simulink model "kalman"  (R2020a)
settings: Solver=VariableStepAuto  StartTime=0.0  StopTime=100  MaxStep=0.01  MinStep=0.01  RelTol=1e-3
model workspace (MAT data in the model file):
  PnFrequencyOffset_26 = [30000 100000 1000000 3000000 10000000]
  uniqueString_26 = '91_3376'
libraries: simulink x1
settings Model: Creator=johan  LastModifiedBy=johan
settings DebuggingCC: UnconnectedInputMsg=none  UnconnectedOutputMsg=none  UnconnectedLineMsg=none
settings ModelReferenceCC: EnableRefExpFcnMdlSchedulingChecks=off
settings RTWCC: Description=Generic Real-Time Target

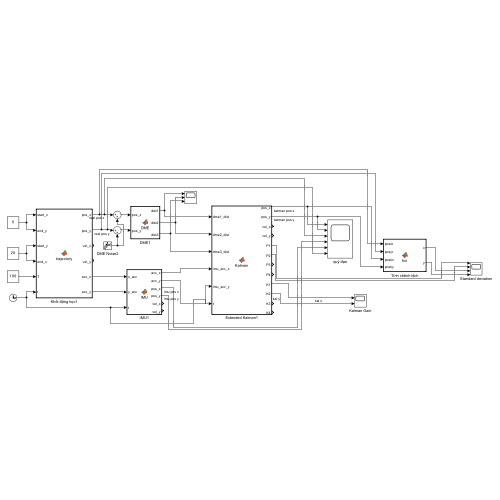
[thumbnail: Simulink's stored preview of the top-level diagram]
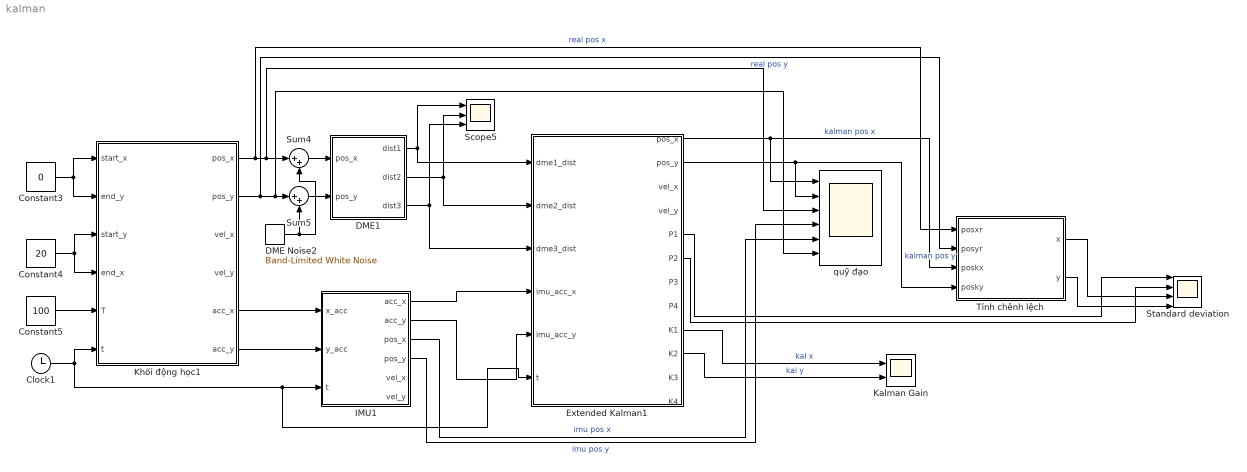
== system kalman ==
  Clock1 : Clock
  Constant3 : Constant  Value=0
  Constant4 : Constant  Value=20
  Constant5 : Constant  Value=100
  DME Noise2 : simulink/Sources/Band-Limited White Noise  Cov=[1e-5]  Ts=0.01  seed=[23341]
  DME1 : MATLAB Function  TreatAsAtomicUnit=on
  Extended Kalman1 : MATLAB Function  TreatAsAtomicUnit=on
  IMU1 : MATLAB Function  TreatAsAtomicUnit=on
  Kalman Gain : Scope  NumInputPorts=2
  Khối động học1 : MATLAB Function  TreatAsAtomicUnit=on
  Scope5 : Scope  NumInputPorts=3
  Standard deviation : Scope  NumInputPorts=4
  Sum4 : Sum  Inputs=|++
  Sum5 : Sum  Inputs=|++
  Tính chênh lệch : MATLAB Function  TreatAsAtomicUnit=on
  quỹ đạo : Scope  NumInputPorts=6
  wires:
  Extended Kalman1/2(pos_y) -> Tính chênh lệch/4(posky), quỹ đạo/2  "kalman pos y"
  Extended Kalman1/1(pos_x) -> Tính chênh lệch/3(poskx), quỹ đạo/1  "kalman pos x"
  Khối động học1/5(acc_x) -> IMU1/1(x_acc)
  IMU1/2(acc_y) -> Extended Kalman1/5(imu_acc_y)
  IMU1/1(acc_x) -> Extended Kalman1/4(imu_acc_x)
  DME1/1(dist1) -> Scope5/1, Extended Kalman1/1(dme1_dist)
  Khối động học1/6(acc_y) -> IMU1/2(y_acc)
  DME1/3(dist3) -> Extended Kalman1/3(dme3_dist), Scope5/3
  DME1/2(dist2) -> Extended Kalman1/2(dme2_dist), Scope5/2
  Constant4/1 -> Khối động học1/3(start_y), Khối động học1/4(end_x)
  Constant5/1 -> Khối động học1/5(T)
  Constant3/1 -> Khối động học1/2(end_y), Khối động học1/1(start_x)
  Clock1/1 -> IMU1/3(t), Extended Kalman1/6(t), Khối động học1/6(t)
  Sum5/1 -> DME1/2(pos_y)
  Sum4/1 -> DME1/1(pos_x)
  DME Noise2/1 -> Sum4/2, Sum5/2
  Khối động học1/2(pos_y) -> Tính chênh lệch/2(posyr), Sum5/1, quỹ đạo/6  "real pos y"
  Khối động học1/1(pos_x) -> Tính chênh lệch/1(posxr), Sum4/1, quỹ đạo/3  "real pos x"
  Extended Kalman1/5(P1) -> Standard deviation/1
  Extended Kalman1/6(P2) -> Standard deviation/2
  IMU1/3(pos_x) -> quỹ đạo/5  "imu pos x"
  IMU1/4(pos_y) -> quỹ đạo/4  "imu pos y"
  Extended Kalman1/9(K1) -> Kalman Gain/1  "kal x"
  Extended Kalman1/10(K2) -> Kalman Gain/2  "kal y"
  Tính chênh lệch/2(y) -> Standard deviation/4
  Tính chênh lệch/1(x) -> Standard deviation/3

== matlab function kalman/Tính chênh lệch ==
  data: x output; posxr input; y output; posyr input; poskx input; posky input
function [x,y] = fcn(posxr, posyr, poskx, posky)
x = abs(posxr-poskx);
y=abs(posyr-posky);

== matlab function kalman/DME1 ==
  data: pos_x input; dist1 output; pos_y input; dist2 output; dist3 output
function [dist1, dist2, dist3] = DME(pos_x, pos_y)
    % Define DME station positions
    dme1_x = 0; dme1_y = 22;     % Position of DME station 1
    dme2_x = 16; dme2_y = 16;      % Position of DME station 2
    dme3_x = 230; dme3_y = 100;     % Position of DME station 3
    
    % Define DME coverage radius
    coverage_radius = 7;
    % Calculate distances to each DME station
    dx1 = pos_x - dme1_x;
    dy1 = pos_y - dme1_y;
    range1 = sqrt(dx1^2 + dy1^2);
    if range1 <= coverage_radius
        dist1 = range1;
    else
        dist1 = NaN;
    end
    
    dx2 = pos_x - dme2_x;
    dy2 = pos_y - dme2_y;
    range2 = sqrt(dx2^2 + dy2^2);
    if range2 <= coverage_radius;
        dist2 = range2;
    else
        dist2 = NaN;
    end
    
    dx3 = pos_x - dme3_x;
    dy3 = pos_y - dme3_y;
    range3 = sqrt(dx3^2 + dy3^2);
    if range3 <= coverage_radius
        dist3 = range3;
    else
        dist3 = NaN;
    end
end

== matlab function kalman/Extended Kalman1 ==
  data: dme1_dist input; dme2_dist input; dme3_dist input; imu_acc_x input; imu_acc_y input; t input; pos_x output; pos_y output; vel_x output; vel_y output; P1 output; P2 output; P3 output; P4 output; K1 output; K2 output; K3 output; K4 output
function [pos_x, pos_y, vel_x, vel_y, P1, P2, P3, P4, K1, K2, K3, K4] = Kalman(dme1_dist, dme2_dist, dme3_dist, imu_acc_x, imu_acc_y, t)

    persistent x_est P_est prev_t
    if isempty(x_est)
        % Initialize state vector [pos_x; pos_y; vel_x; vel_y]
        x_est = [0; 20; 0; 0];  % Initial position 
        P_est = eye(4) * 1e-30;      % Initial state covariance
        prev_t = 0;
    end
    
    % Calculate dt
    dt = t - prev_t;
    prev_t = t; 
    a=2e-5;
    b=1.9e-5;
    c = 0;
    % Process noise covariance (Q)
    Q = [a	c  0	0;
          c   b	  0	0;
            0	        0	      0	0;
            0          0	      0	0];  
    
    R_single = 9.8e-04;  % Measurement noise variance
    
    % DME station positions
    dme1_pos = [0, 22];   % DME 1
    dme2_pos = [16, 16];  % DME 2
    dme3_pos = [23, 0];  % DME 3
    
    % Prediction Step
    % State transition matrix (F)
    F = [1, 0, dt, 0;
         0, 1, 0, dt;
         0, 0, 1, 0;
         0, 0, 0, 1];
    
    % Input matrix (B) for acceleration
    B = [0.5*dt^2, 0;
         0, 0.5*dt^2;
         dt, 0;
         0, dt];
    
    % Predict state
    x_pred = F * x_est + B * [imu_acc_x; imu_acc_y];
    
    % Predict covariance
    P_pred = F * P_est * F' + Q;
    
    % Update Step
    % Initialize measurement matrices
    H = zeros(1, 4);  % Single measurement, 4 states
    z = 0;            % Valid measurement
    h_x = 0;          % Predicted measurement
    R = 0;            % Measurement noise covariance
    
    % Check DME 1
    if dme1_dist > 0  % Valid measurement
        dx = x_pred(1) - dme1_pos(1);
        dy = x_pred(2) - dme1_pos(2);
        dist = sqrt(dx^2 + dy^2);
        
        % Populate H, z, h_x, and R for DME 1
        H = [dx/dist, dy/dist, 0, 0];
        z = dme1_dist;
        h_x = dist;
        R = R_single;
    end
    
    % Check DME 2
    if dme2_dist > 0  % Valid measurement
        dx = x_pred(1) - dme2_pos(1);
        dy = x_pred(2) - dme2_pos(2);
        dist = sqrt(dx^2 + dy^2);
        
        % Populate H, z, h_x, and R for DME 2
        H = [dx/dist, dy/dist, 0, 0];
        z = dme2_dist;
        h_x = dist;
        R = R_single;
    end
    
    % Check DME 3
    if dme3_dist > 0  % Valid measurement
        dx = x_pred(1) - dme3_pos(1);
        dy = x_pred(2) - dme3_pos(2);
        dist = sqrt(dx^2 + dy^2);
        
        % Populate H, z, h_x, and R for DME 3
        H = [dx/dist, dy/dist, 0, 0];
        z = dme3_dist;
        h_x = dist;
        R = R_single;
    end
    
    % Update state if we have a valid measurement
    if R > 0
        % Calculate Kalman gain
        S = H * P_pred * H' + R;
        K = P_pred * H' / S;
        
        % Extract components of Kalman gain
        K1 = K(1);
        K2 = K(2);
        K3 = K(3);
        K4 = K(4);
        
        % Update state and covariance
        residual = z - h_x;
        x_est = x_pred + K * residual;
        P_est = (eye(4) - K * H) * P_pred;
    else
        % If no valid measurements, use prediction
        x_est = x_pred;
        P_est = P_pred;
        K1 = 0;
        K2 = 0;
        K3 = 0;
        K4 = 0;
    end
        P1 = sqrt(P_est(1,1));
        P2 = sqrt(P_est(2,2));
            P3 = sqrt(P_est(3,3));
                P4 = sqrt(P_est(4,4));
    % Output estimated states and Kalman gain components
    pos_x = x_est(1);
    pos_y = x_est(2);
    vel_x = x_est(3);
    vel_y = x_est(4);
end

== matlab function kalman/IMU1 ==
  data: acc_x output; acc_y output; x_acc input; pos_x output; y_acc input; t input; pos_y output; vel_x output; vel_y output
function [ acc_x, acc_y,pos_x, pos_y, vel_x, vel_y] = IMU(x_acc, y_acc, t)
    g = 9.81;  % gravity constant [m/s^2]
    persistent prev_vel_x prev_vel_y prev_pos_x prev_pos_y prev_t
   
    if isempty(prev_vel_x)
        prev_vel_x = 0;
        prev_vel_y = 0;
        prev_pos_x = 0;  % Set to match trajectory starting position
        prev_pos_y = 20;  % Set to match trajectory starting position
        prev_t = 0;
    end
    
    % Calculate dt
    dt = t - prev_t;
    
    % Error parameters
    acc_bias_mps2 = 1e-5 * 9.81;  % accelerometer bias
    gyro_bias_rps = 1e-3 * (pi/180) / 3600;  % gyroscope bias
    init_heading_error_rad =1e-5 * (pi/180);  % heading error
    init_velocity_error = 0;  % velocity error
    init_position_error = 0;  % position error
    
    % Calculate errors 
    delta_theta = init_heading_error_rad + gyro_bias_rps * t;
    
    delta_v = init_velocity_error + acc_bias_mps2 * t - ...
              g * init_heading_error_rad * t - ...
              g * gyro_bias_rps * t^2;
    
    delta_p = init_position_error + init_velocity_error * t + ...
              0.5 * acc_bias_mps2 * t^2 - ...
              0.5 * g * init_heading_error_rad * t^2 - ...
              (1/6) * g * gyro_bias_rps * t^3;
    
    % Add bias to accelerometer readings
    acc_x = x_acc + acc_bias_mps2;
    acc_y = y_acc + acc_bias_mps2;
    
    % Integrate acceleration to get velocity
    vel_x = prev_vel_x + acc_x * dt;
    vel_y = prev_vel_y + acc_y * dt;
    
    % Add velocity error
    vel_x = vel_x + delta_v;
    vel_y = vel_y + delta_v;
    
    % Integrate velocity to get position
    pos_x = prev_pos_x + prev_vel_x * dt + 0.5 * acc_x * dt * dt;  
    pos_y = prev_pos_y + prev_vel_y * dt + 0.5 * acc_y * dt * dt;
    
    % Add position error
    pos_x = pos_x + delta_p;
    pos_y = pos_y + delta_p;
    
    % Update persistent variables
    prev_vel_x = vel_x - delta_v;
    prev_vel_y = vel_y - delta_v;
    prev_pos_x = pos_x - delta_p;
    prev_pos_y = pos_y - delta_p;
    prev_t = t;

end

== matlab function kalman/Khối động học1 ==
  data: start_x input; end_y input; start_y input; end_x input; T input; t input; pos_x output; pos_y output; vel_x output; vel_y output; acc_x output; acc_y output
function [pos_x, pos_y, vel_x, vel_y, acc_x, acc_y] = trajectory( start_x, end_y, start_y, end_x, T,t)
    % Normalize time to [0,1]
    t_norm = t/T;
    if t_norm > 1
        t_norm = 1;
    end
    
% X-direction
a0 = 0; a1 = 0; a2 = 0; a3 = 10; a4 = -15; a5 = 6;
% Y-direction
b0 = 0; b1 = 0; b2 = 0; b3 = 9; b4 = -18; b5 = 10;

    % Calculate normalized position 
    s = a0 + a1*t_norm + a2*t_norm^2 + a3*t_norm^3 + a4*t_norm^4 + a5*t_norm^5;
    
    % Calculate normalized velocity
    s_dot = (a1 + 2*a2*t_norm + 3*a3*t_norm^2 + 4*a4*t_norm^3 + 5*a5*t_norm^4)/T;
    
    % Calculate normalized acceleration
    s_ddot = (2*a2 + 6*a3*t_norm + 12*a4*t_norm^2 + 20*a5*t_norm^3)/T^2;
    
        % Calculate normalized position 
    s2 = b0 + b1*t_norm + b2*t_norm^2 + b3*t_norm^3 + b4*t_norm^4 + b5*t_norm^5;
    
    % Calculate normalized velocity
    s_dot2 = (b1 + 2*b2*t_norm + 3*b3*t_norm^2 + 4*b4*t_norm^3 + 5*b5*t_norm^4)/T;
    
    % Calculate normalized acceleration
    s_ddot2 = (2*b2 + 6*b3*t_norm + 12*b4*t_norm^2 + 20*b5*t_norm^3)/T^2;
    
    % Calculate actual positions
    pos_x = start_x + (end_x - start_x) * s;
    pos_y = start_y + (end_y - start_y) * s2;
    
    % Calculate actual velocities
    vel_x = (end_x - start_x) * s_dot;
    vel_y = (end_y - start_y) * s_dot2;
    
    % Calculate actual accelerations
    acc_x = (end_x - start_x) * s_ddot;
    acc_y = (end_y - start_y) * s_ddot2;
end
